simulink model "kalman_sim_K"  (R2017b)
settings: Solver=VariableStepAuto  StartTime=0.0  StopTime=2000  FixedStep=5  RelTol=1e-3
values from neighbouring files (symbols this model uses):
  A = [A11 A12 A13 A14; A21 A22 A23 A24; A31 A32 A33 A34; A41 A42 A43 A44]    [oneforall.m]
  B = [0;0;0;1/jm]    [oneforall.m]
  C = eye(4)    [oneforall.m]
  K = 12    [TD6.m]    (also in oneforall.m = place(A,B,P))
  M = [0.1 0 0 0; 0 0.1 0 0; 0 0 0.00132 0 ;0 0 0 0.1]    [oneforall.m]
undefined symbols (not defined in the file or in its folder): Kf
libraries: simulink x3
settings Model: Creator=lencs  LastModifiedBy=lencs

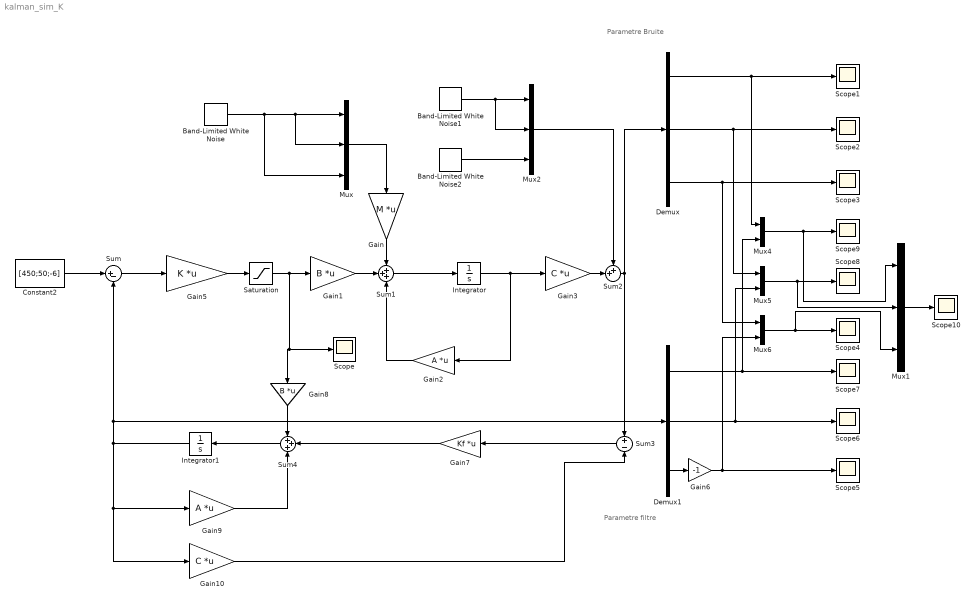
== system kalman_sim_K ==
  note: Parametre Bruite
  note: Parametre filtre
  Band-Limited White Noise : simulink/Sources/Band-Limited White Noise  Cov=[0.05]  Ts=0.5  seed=[23341]
  Band-Limited White Noise1 : simulink/Sources/Band-Limited White Noise  Cov=[0.05]  Ts=0.5  seed=[23341]
  Band-Limited White Noise2 : simulink/Sources/Band-Limited White Noise  Cov=[0.05]  Ts=0.5  seed=[23341]
  Constant2 : Constant  Value=[450;50;-6]
  Demux : Demux  Outputs=3
  Demux1 : Demux  Outputs=3
  Gain : Gain  Gain=M  Multiplication=Matrix(K*u) (u vector)
  Gain1 : Gain  Gain=B  Multiplication=Matrix(K*u) (u vector)
  Gain10 : Gain  Gain=C  Multiplication=Matrix(K*u) (u vector)
  Gain2 : Gain  Gain=A  Multiplication=Matrix(K*u)
  Gain3 : Gain  Gain=C  Multiplication=Matrix(K*u) (u vector)
  Gain5 : Gain  Gain=K  Multiplication=Matrix(K*u) (u vector)
  Gain6 : Gain  Gain=-1
  Gain7 : Gain  Gain=Kf  Multiplication=Matrix(K*u)
  Gain8 : Gain  Gain=B  Multiplication=Matrix(K*u)
  Gain9 : Gain  Gain=A  Multiplication=Matrix(K*u) (u vector)
  Integrator : Integrator  InitialCondition=[200; 30; -30]
  Integrator1 : Integrator
  Mux : Mux  Inputs=3
  Mux1 : Mux  Inputs=3
  Mux2 : Mux  Inputs=3
  Mux4 : Mux  Inputs=2
  Mux5 : Mux  Inputs=2
  Mux6 : Mux  Inputs=2
  Saturation : Saturate  UpperLimit=pi/2  LowerLimit=0
  Scope{,1..10} (11 alike) : Scope
  Sum : Sum  Inputs=|+-
  Sum1 : Sum  Inputs=+++
  Sum2 : Sum  Inputs=++|
  Sum3 : Sum  Inputs=+-
  Sum4 : Sum  Inputs=+++
  wires:
  Band-Limited White Noise/1 -> Mux/3, Mux/2, Mux/1
  Mux/1 -> Gain/1
  Constant2/1 -> Sum/1
  Saturation/1 -> Scope/1, Gain8/1, Gain1/1
  Gain1/1 -> Sum1/2
  Gain/1 -> Sum1/1
  Sum1/1 -> Integrator/1
  Integrator/1 -> Gain2/1, Gain3/1
  Demux/2 -> Mux5/1, Scope2/1
  Gain2/1 -> Sum1/3
  Sum/1 -> Gain5/1
  Gain5/1 -> Saturation/1
  Demux/3 -> Mux6/1, Scope3/1
  Gain3/1 -> Sum2/2
  Sum2/1 -> Demux/1, Sum3/1
  Mux2/1 -> Sum2/1
  Band-Limited White Noise1/1 -> Mux2/2, Mux2/1
  Band-Limited White Noise2/1 -> Mux2/3
  Demux1/3 -> Gain6/1
  Sum3/1 -> Gain7/1
  Gain7/1 -> Sum4/2
  Gain8/1 -> Sum4/1
  Sum4/1 -> Integrator1/1
  Integrator1/1 -> Sum/2, Demux1/1, Gain10/1, Gain9/1
  Gain9/1 -> Sum4/3
  Gain10/1 -> Sum3/2
  Demux1/2 -> Mux5/2, Scope6/1
  Gain6/1 -> Mux6/2, Scope5/1
  Demux1/1 -> Mux4/2, Scope7/1
  Mux6/1 -> Mux1/3, Scope4/1
  Mux5/1 -> Mux1/2, Scope8/1
  Mux4/1 -> Mux1/1, Scope9/1
  Demux/1 -> Mux4/1, Scope1/1
  Mux1/1 -> Scope10/1
